simulink model "Modeling_Control"  (R2023b)
settings: Solver=VariableStepAuto  StartTime=0.0  StopTime=500  RelTol=1e-3
values from neighbouring files (symbols this model uses):
  k = 1    [SystemModeling.m]
undefined symbols (not defined in the file or in its folder): g, M1, M2, mu
libraries: slpidlib x1, SignalEditorBlockLib x1
settings Model: Creator=lee  LastModifiedBy=lee

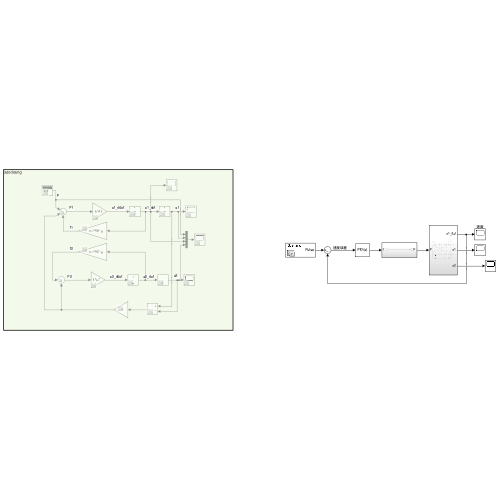
[thumbnail: Simulink's stored preview of the top-level diagram]
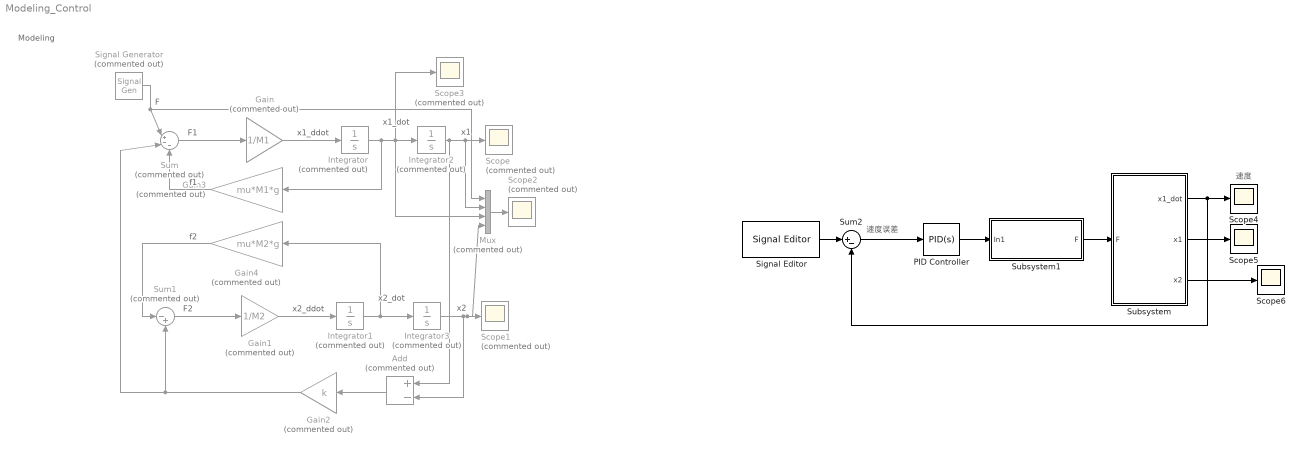
== system Modeling_Control ==
  note: 速度误差
  note: 速度
  note: Modeling
  note: f2
  note: F
  note: x1
  note: x1_dot
  note: x1_ddot
  note: F1
  note: F2
  note: x2_ddot
  note: x2_dot
  note: x2
  note: f1
  Add : Sum  Commented=on  Inputs=+-
  Gain : Gain  Commented=on  Gain=1/M1
  Gain1 : Gain  Commented=on  Gain=1/M2
  Gain2 : Gain  Commented=on  Gain=k
  Gain3 : Gain  Commented=on  Gain=mu*M1*g
  Gain4 : Gain  Commented=on  Gain=mu*M2*g
  Integrator{,1..3} (4 alike) : Integrator  Commented=on
  Mux : Mux  Commented=on
  PID Controller : slpidlib/PID Controller  Controller=PID  Form=Parallel  TimeDomain=Continuous-time  UseExternalTs=off  SampleTime=-1  IntegratorMethod=Forward Euler  FilterMethod=Forward Euler  ControllerParametersSource=internal  P=1.06928582106373  I=0.19504989406495  UseKiTs=off  D=-0.0883512602923273  N=3.57228246989798  UseFilter=on  TunerSelectOption=Transfer Function Based (PID Tuner App)  InitialConditionSource=internal  InitialConditionForIntegrator=0  InitialConditionForFilter=0  DifferentiatorICPrevScaledInput=0  ExternalReset=none  TrackingMode=off  Kt=1  LimitOutput=off  SatLimitsSource=internal  UpperSaturationLimit=inf  LowerSaturationLimit=-inf  LinearizeAsGain=on  AntiWindupMode=none  Kb=1  LimitIntegrator=off  UpperIntegratorSaturationLimit=inf  LowerIntegratorSaturationLimit=-inf  POutMin=[]  POutMax=[]  IOutMin=[]  IOutMax=[]  DOutMin=[]  DOutMax=[]  NOutMin=[]  NOutMax=[]  SumOutMin=[]  SumOutMax=[]  SaturationOutMin=[]  SaturationOutMax=[]  PParamMin=[]  PParamMax=[]  IParamMin=[]  IParamMax=[]  DParamMin=[]  DParamMax=[]  NParamMin=[]  NParamMax=[]  KbParamMin=[]  KbParamMax=[]  KtParamMin=[]  KtParamMax=[]  KbOutMin=[]  KbOutMax=[]  KtOutMin=[]  KtOutMax=[]  IntegratorOutMin=[]  IntegratorOutMax=[]  FilterOutMin=[]  FilterOutMax=[]  SumI1OutMin=[]  SumI1OutMax=[]  SumI2OutMin=[]  SumI2OutMax=[]  SumI3OutMin=[]  SumI3OutMax=[]  SumI4OutMin=[]  SumI4OutMax=[]  SumDOutMin=[]  SumDOutMax=[]  DifferentiatorOutMin=[]  DifferentiatorOutMax=[]  FilterDiffOutCoefMin=[]  FilterDiffOutCoefMax=[]  ReciprocalOutMin=[]  ReciprocalOutMax=[]  SumDenOutMin=[]  SumDenOutMax=[]  SumNumOutMin=[]  SumNumOutMax=[]  DivideOutMin=[]  DivideOutMax=[]  UdiffTsProdOutMin=[]  UdiffTsProdOutMax=[]  NTsProdOutMin=[]  NTsProdOutMax=[]  UintegralTsProdOutMin=[]  UintegralTsProdOutMax=[]  UngainTsProdOutMin=[]  UngainTsProdOutMax=[]  ClampingZeroOutDataTypeStr=Inherit: Inherit via back propagation  ClampingZeroOutMin=[]  ClampingZeroOutMax=[]  FilterDenConstantOutDataTypeStr=Inherit: Inherit via back propagation  FilterDenConstantOutMin=[]  FilterDenConstantOutMax=[]  PCopyOutDataTypeStr=Inherit: Inherit via back propagation  PCopyOutMin=[]  PCopyOutMax=[]  NCopyOutDataTypeStr=Inherit: Inherit via back propagation  NCopyOutMin=[]  NCopyOutMax=[]  IntegratorContinuousStateAttributes=''  IntegratorStateMustResolveToSignalObject=off  IntegratorRTWStateStorageClass=Auto  FilterContinuousStateAttributes=''  FilterStateMustResolveToSignalObject=off  FilterRTWStateStorageClass=Auto  ParallelPVariant=InternalParameters  IdealPVariant=Disabled  IVariant=InternalParameters  DVariant=InternalParameters  IntegratorVariant=Continuous  SatVariant=Disabled  AWVariant=Passthrough  PCopyVariant=Disabled  TRVariant=Disabled  FdbkBlocksVariant=Forward  IdealPFdbkVariant=Disabled  SatFdbkVariant=Disabled  DerivativeFilterVariant=ContFilter  NVariant=InternalParameters  NCopyVariant=Disabled  FilterICVariant=InternalICsFilter  IntegratorICVariant=InternalICs  ExternalResetVariant=Disabled  TRSumVariant=Passthrough  SumFdbkVariant=Disabled  SumVariant=Sum_PID  TsampFilterVariant=InternalTs  TsampNgainVariant=Passthrough  TsampIntegralVariant=Disabled_SignalSpec  ExternalSaturationOutDataTypeStr=Inherit: Same as second input
  Scope{,1..3} (4 alike) : Scope  Commented=on
  Scope4 : Scope
  Scope5 : Scope
  Scope6 : Scope
  Signal Generator : SignalGenerator  Commented=on  WaveForm=square  Amplitude=-1  Frequency=0.001
  Signal Editor : SignalEditorBlockLib/Signal Editor  FileName=train.mat  ActiveScenario=Scenario  ActiveSignal=Pulse  IsBus=off  OutputBusObjectStr=Bus: BusObject  SampleTime=0  Interpolate=off  ZeroCross=off  OutputAfterFinalValue=Setting to zero  Unit=inherit  PreserveSignalName=on  ApplySigPropsToAllScenarios=on  ApplySigPropsToAllSignals=off
  Subsystem : Subsystem
  Subsystem1 : Subsystem
  Sum : Sum  Commented=on  Inputs=|+--
  Sum1 : Sum  Commented=on  Inputs=|-+
  Sum2 : Sum  Inputs=|+-
  wires:
  Sum/1 -> Gain/1
  Sum1/1 -> Gain1/1
  Gain/1 -> Integrator/1
  Gain1/1 -> Integrator1/1
  Integrator/1 -> Gain3/1, Scope3/1, Mux/3, Integrator2/1
  Integrator1/1 -> Gain4/1, Integrator3/1
  Integrator2/1 -> Mux/2, Scope/1, Add/1
  Integrator3/1 -> Mux/4, Scope1/1, Add/2
  Signal Generator/1 -> Mux/1, Sum/1
  Add/1 -> Gain2/1
  Gain2/1 -> Sum/2, Sum1/2
  Gain3/1 -> Sum/3
  Gain4/1 -> Sum1/1
  Mux/1 -> Scope2/1
  Subsystem/1(x1_dot) -> Scope4/1, Sum2/2
  Subsystem/2(x1) -> Scope5/1
  Subsystem/3(x2) -> Scope6/1
  Subsystem1/1(F) -> Subsystem/1(F)
  PID Controller/1 -> Subsystem1/1(In1)
  Sum2/1 -> PID Controller/1
  Signal Editor/1 -> Sum2/1

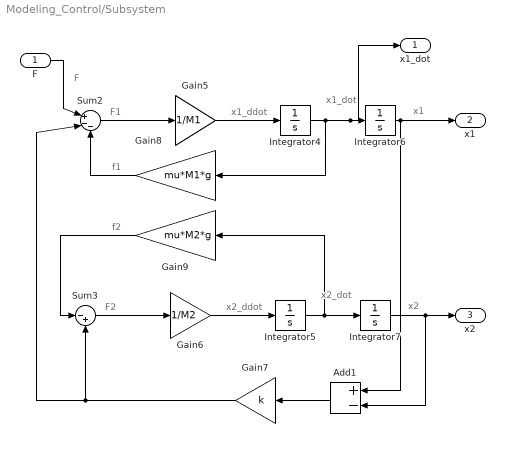
== system Modeling_Control/Subsystem ==
  note: x2_dot
  note: x1_ddot
  note: f1
  note: x2
  note: x1_dot
  note: x2_ddot
  note: F1
  note: F
  note: F2
  note: f2
  note: x1
  F : Inport
  Add1 : Sum  Inputs=+-
  Gain5 : Gain  Gain=1/M1
  Gain6 : Gain  Gain=1/M2
  Gain7 : Gain  Gain=k
  Gain8 : Gain  Gain=mu*M1*g
  Gain9 : Gain  Gain=mu*M2*g
  Integrator{4..7} (4 alike) : Integrator
  Sum2 : Sum  Inputs=|+--
  Sum3 : Sum  Inputs=|-+
  x1_dot : Outport
  x1 : Outport  Port=2
  x2 : Outport  Port=3
  wires:
  F/1 -> Sum2/1
  Gain6/1 -> Integrator5/1
  Add1/1 -> Gain7/1
  Sum3/1 -> Gain6/1
  Gain5/1 -> Integrator4/1
  Integrator5/1 -> Gain9/1, Integrator7/1
  Integrator6/1 -> x1/1, Add1/1
  Sum2/1 -> Gain5/1
  Gain8/1 -> Sum2/3
  Gain9/1 -> Sum3/1
  Integrator7/1 -> x2/1, Add1/2
  Integrator4/1 -> Gain8/1, x1_dot/1, Integrator6/1
  Gain7/1 -> Sum2/2, Sum3/2

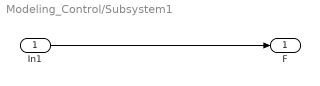
== system Modeling_Control/Subsystem1 ==
  In1 : Inport
  F : Outport
  wires:
  In1/1 -> F/1
